simulink model "MPModel_FeedforwardNetwork_4GL"  (R2015a)
settings: Solver=ode3  StartTime=0.0  StopTime=5  FixedStep=0.01  RelTol=1e-3
settings Model: Creator=Admin  LastModifiedBy=Sneha More
settings DataIOCC: LimitDataPoints=off
settings DebuggingCC: UnderspecifiedInitializationDetection=Classic  MergeDetectMultiDrivingBlocksExec=none  SolverPrmCheckMsg=warning  StateNameClashWarn=warning

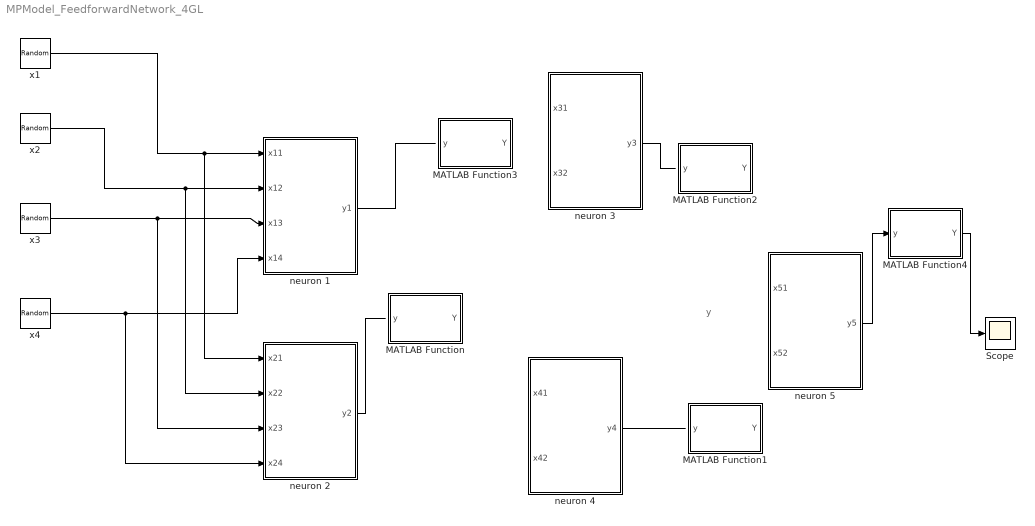
== system MPModel_FeedforwardNetwork_4GL ==
  note: y
  MATLAB Function : MATLAB Function  TreatAsAtomicUnit=on
  MATLAB Function1 : MATLAB Function  TreatAsAtomicUnit=on
  MATLAB Function2 : MATLAB Function  TreatAsAtomicUnit=on
  MATLAB Function3 : MATLAB Function  TreatAsAtomicUnit=on
  MATLAB Function4 : MATLAB Function  TreatAsAtomicUnit=on
  Scope : Scope
      settings: SaveName=yk
  neuron 1 : Subsystem
  neuron 2 : Subsystem
  neuron 3 : Subsystem
  neuron 4 : Subsystem
  neuron 5 : Subsystem
  x{1..4} (4 alike) : RandomNumber
  wires:
  x4/1 -> neuron 2/4(x24), neuron 1/4(x14)
  x1/1 -> neuron 2/1(x21), neuron 1/1(x11)
  x2/1 -> neuron 2/2(x22), neuron 1/2(x12)
  x3/1 -> neuron 2/3(x23), neuron 1/3(x13)
  neuron 1/1(y1) -> ?
  ? -> neuron 4/1(x41), neuron 3/1(x31)
  neuron 2/1(y2) -> ?
  ? -> neuron 4/2(x42), neuron 3/2(x32)
  neuron 3/1(y3) -> ?
  ? -> neuron 5/1(x51)
  neuron 4/1(y4) -> ?
  ? -> neuron 5/2(x52)
  neuron 5/1(y5) -> MATLAB Function4/1(y)
  MATLAB Function4/1(Y) -> Scope/1

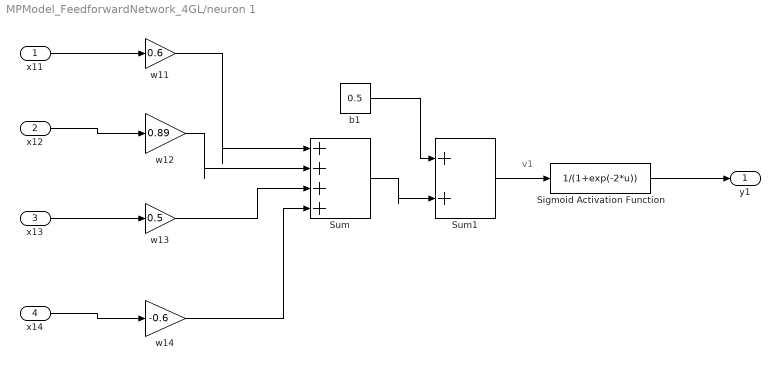
== system MPModel_FeedforwardNetwork_4GL/neuron 1 ==
  note: v1
  x11 : Inport
  x12 : Inport  Port=2
  x13 : Inport  Port=3
  x14 : Inport  Port=4
  Sigmoid Activation Function : Fcn  Expr=1/(1+exp(-2*u))
  Sum : Sum  Inputs=|++++
  Sum1 : Sum  Inputs=|++
  b1 : Constant  Value=0.5
  w11 : Gain  Gain=0.6
  w12 : Gain  Gain=0.89
  w13 : Gain  Gain=0.5
  w14 : Gain  Gain=-0.6
  y1 : Outport
  wires:
  Sum1/1 -> Sigmoid Activation Function/1
  Sum/1 -> Sum1/2
  Sigmoid Activation Function/1 -> y1/1
  b1/1 -> Sum1/1
  x11/1 -> w11/1
  w11/1 -> Sum/1
  x14/1 -> w14/1
  w14/1 -> Sum/4
  w13/1 -> Sum/3
  x12/1 -> w12/1
  w12/1 -> Sum/2
  x13/1 -> w13/1

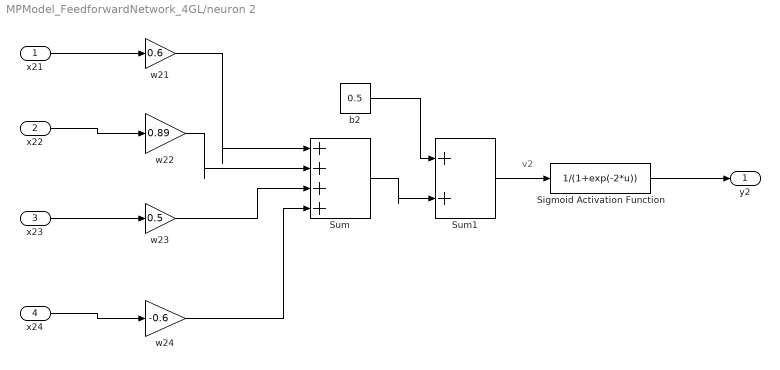
== system MPModel_FeedforwardNetwork_4GL/neuron 2 ==
  note: v2
  x21 : Inport
  x22 : Inport  Port=2
  x23 : Inport  Port=3
  x24 : Inport  Port=4
  Sigmoid Activation Function : Fcn  Expr=1/(1+exp(-2*u))
  Sum : Sum  Inputs=|++++
  Sum1 : Sum  Inputs=|++
  b2 : Constant  Value=0.5
  w21 : Gain  Gain=0.6
  w22 : Gain  Gain=0.89
  w23 : Gain  Gain=0.5
  w24 : Gain  Gain=-0.6
  y2 : Outport
  wires:
  Sum1/1 -> Sigmoid Activation Function/1
  Sum/1 -> Sum1/2
  Sigmoid Activation Function/1 -> y2/1
  b2/1 -> Sum1/1
  x21/1 -> w21/1
  w21/1 -> Sum/1
  x24/1 -> w24/1
  w24/1 -> Sum/4
  w23/1 -> Sum/3
  x22/1 -> w22/1
  w22/1 -> Sum/2
  x23/1 -> w23/1

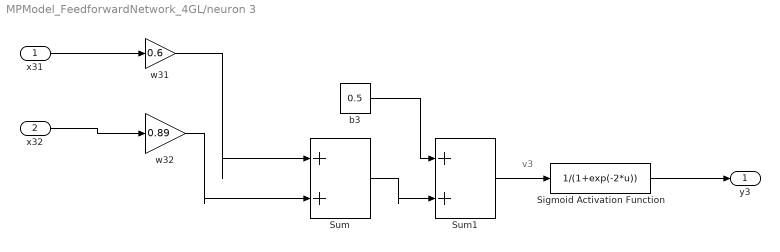
== system MPModel_FeedforwardNetwork_4GL/neuron 3 ==
  note: v3
  x31 : Inport
  x32 : Inport  Port=2
  Sigmoid Activation Function : Fcn  Expr=1/(1+exp(-2*u))
  Sum : Sum  Inputs=|++
  Sum1 : Sum  Inputs=|++
  b3 : Constant  Value=0.5
  w31 : Gain  Gain=0.6
  w32 : Gain  Gain=0.89
  y3 : Outport
  wires:
  w32/1 -> Sum/2
  x32/1 -> w32/1
  w31/1 -> Sum/1
  x31/1 -> w31/1
  b3/1 -> Sum1/1
  Sigmoid Activation Function/1 -> y3/1
  Sum/1 -> Sum1/2
  Sum1/1 -> Sigmoid Activation Function/1

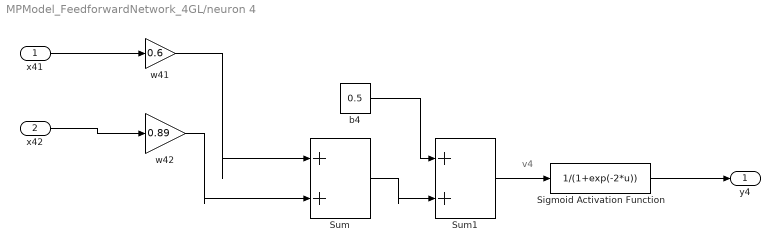
== system MPModel_FeedforwardNetwork_4GL/neuron 4 ==
  note: v4
  x41 : Inport
  x42 : Inport  Port=2
  Sigmoid Activation Function : Fcn  Expr=1/(1+exp(-2*u))
  Sum : Sum  Inputs=|++
  Sum1 : Sum  Inputs=|++
  b4 : Constant  Value=0.5
  w41 : Gain  Gain=0.6
  w42 : Gain  Gain=0.89
  y4 : Outport
  wires:
  Sum1/1 -> Sigmoid Activation Function/1
  Sum/1 -> Sum1/2
  Sigmoid Activation Function/1 -> y4/1
  b4/1 -> Sum1/1
  x41/1 -> w41/1
  w41/1 -> Sum/1
  x42/1 -> w42/1
  w42/1 -> Sum/2

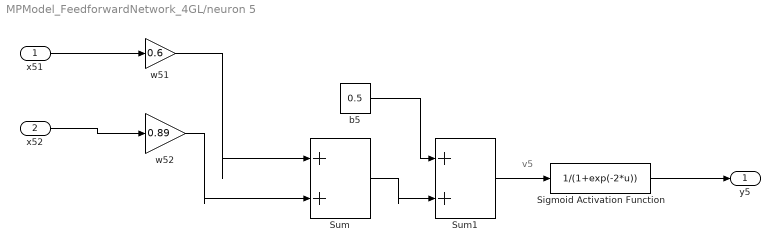
== system MPModel_FeedforwardNetwork_4GL/neuron 5 ==
  note: v5
  x51 : Inport
  x52 : Inport  Port=2
  Sigmoid Activation Function : Fcn  Expr=1/(1+exp(-2*u))
  Sum : Sum  Inputs=|++
  Sum1 : Sum  Inputs=|++
  b5 : Constant  Value=0.5
  w51 : Gain  Gain=0.6
  w52 : Gain  Gain=0.89
  y5 : Outport
  wires:
  w52/1 -> Sum/2
  x52/1 -> w52/1
  w51/1 -> Sum/1
  x51/1 -> w51/1
  b5/1 -> Sum1/1
  Sigmoid Activation Function/1 -> y5/1
  Sum/1 -> Sum1/2
  Sum1/1 -> Sigmoid Activation Function/1

== matlab function MPModel_FeedforwardNetwork_4GL/MATLAB Function1 ==
  data: y input; Y output
function Y = fgl_deriv1( y )
%#codegen
a=0.5;
h= 0.01;
 n  = numel(y);
    J  = 0:(n-1);
    G1 = gamma( J+1 );
    G2 = gamma( a+1-J );
    s  = (-1) .^ J;

    M  = tril( ones(n) );
    R  = toeplitz( y(:)' );
    T  = meshgrid( (gamma(a+1)/(h^a)) * s ./ (G1.*G2) );
    Y  = reshape(sum( R .* M .* T, 2 ), size(y));
    
    
end

== matlab function MPModel_FeedforwardNetwork_4GL/MATLAB Function ==
  data: y input; Y output
function Y = fgl_deriv( y )
%#codegen
a=0.5;
h= 0.01;
 n  = numel(y);
    J  = 0:(n-1);
    G1 = gamma( J+1 );
    G2 = gamma( a+1-J );
    s  = (-1) .^ J;

    M  = tril( ones(n) );
    R  = toeplitz( y(:)' );
    T  = meshgrid( (gamma(a+1)/(h^a)) * s ./ (G1.*G2) );
    Y  = reshape(sum( R .* M .* T, 2 ), size(y));
    
    
end

== matlab function MPModel_FeedforwardNetwork_4GL/MATLAB Function2 ==
  data: y input; Y output
function Y = fgl_deriv2( y )
%#codegen
a=0.5;
h= 0.01;
 n  = numel(y);
    J  = 0:(n-1);
    G1 = gamma( J+1 );
    G2 = gamma( a+1-J );
    s  = (-1) .^ J;

    M  = tril( ones(n) );
    R  = toeplitz( y(:)' );
    T  = meshgrid( (gamma(a+1)/(h^a)) * s ./ (G1.*G2) );
    Y  = reshape(sum( R .* M .* T, 2 ), size(y));
    
    
end

== matlab function MPModel_FeedforwardNetwork_4GL/MATLAB Function3 ==
  data: y input; Y output
function Y = fgl_deriv3( y )
%#codegen
a=0.5;
h= 0.01;
 n  = numel(y);
    J  = 0:(n-1);
    G1 = gamma( J+1 );
    G2 = gamma( a+1-J );
    s  = (-1) .^ J;

    M  = tril( ones(n) );
    R  = toeplitz( y(:)' );
    T  = meshgrid( (gamma(a+1)/(h^a)) * s ./ (G1.*G2) );
    Y  = reshape(sum( R .* M .* T, 2 ), size(y));
    
    
end

== matlab function MPModel_FeedforwardNetwork_4GL/MATLAB Function4 ==
  data: y input; Y output
function Y = fgl_deriv4( y )
%#codegen
a=0.5;
h= 0.01;
 n  = numel(y);
    J  = 0:(n-1);
    G1 = gamma( J+1 );
    G2 = gamma( a+1-J );
    s  = (-1) .^ J;

    M  = tril( ones(n) );
    R  = toeplitz( y(:)' );
    T  = meshgrid( (gamma(a+1)/(h^a)) * s ./ (G1.*G2) );
    Y  = reshape(sum( R .* M .* T, 2 ), size(y));
    
    
end
